simulink model "px4log"  (R2021a)
settings: Solver=FixedStepAuto  StartTime=0.0  StopTime=inf  RelTol=1e-3  EnableMultiTasking=on
model workspace (MAT data in the model file):
  Ts = 0.01
values from neighbouring files (symbols this model uses):
  den_lpf_d = den_lpf20    [Mainframe_init.m]    (also in load_autopilot.m)
  num_lpf_d = num_lpf20    [Mainframe_init.m]    (also in load_autopilot.m)
undefined symbols (not defined in the file or in its folder): Autopilot, AUX, dev, DiscIntNeverNeededParam, HIL_Data, pwm_output1, x, y, z
libraries: px4uORBlib x6, simulink_extras x4, px4Sensorslib x3, px4lib x2, simulink x1, sharedtransform x1
settings Model: SimulationMode=external  ExtModeTrigDuration=10  Creator=WrySi  LastModifiedBy=sasson
settings SolverCC: AlgebraicLoopSolver=TrustRegion  PositivePriorityOrder=on
settings DataIOCC: MaxDataPoints=2000
settings OptimizationCC: EnhancedBackFolding=on  PassReuseOutputArgsAs=Individual arguments  ZeroExternalMemoryAtStartup=off  ZeroInternalMemoryAtStartup=off  MaxStackSize=64  OptimizeBlockOrder=speed  DifferentSizesBufferReuse=on  OptimizationCustomize=off  EfficientTunableParamExpr=on
settings DebuggingCC: MultiTaskRateTransMsg=warning  ParameterOverflowMsg=none  ParameterTunabilityLossMsg=error  SymbolicDimsDataTypeCodeGenerationDiagnostic=none  SFMachineParentedDataDiag=warning
settings HardwareCC: ProdBitPerPointer=32  ProdBitPerSizeT=32  ProdBitPerPtrDiffT=32  ProdLargestAtomicInteger=Long  ProdLargestAtomicFloat=Double  ProdWordSize=32  ProdLongLongMode=on  ProdHWDeviceType=ARM Compatible->ARM Cortex
settings SFSimCC: MATLABDynamicMemAlloc=off  SimTargetLang=C++
settings RTWCC: SystemTargetFile=ert.tlc  HardwareBoard=PX4 Pixhawk 2.1 (Cube)  TLCOptions="-aInlineSetEventsForThisBaseRateFcn=TLC_FALSE -aSuppressMultiTaskScheduler=TLC_FALSE  -aRateBasedStepFcn=0"  TemplateMakefile=ert_default_tmf  GenerateReport=on  Toolchain=GNU Tools for PX4 Autopilots  IncludeHyperlinkInReport=on  LaunchReport=on  TargetLang=C++  GenerateTraceInfo=on  GenerateTraceReport=on  GenerateTraceReportSl=on  GenerateTraceReportSf=on  GenerateTraceReportEml=on
settings CodeAppCC: ForceParamTrailComments=on  IgnoreCustomStorageClasses=off  OperatorAnnotations=on  SimulinkDataObjDesc=on  SFDataObjDesc=on  InsertBlockDesc=on
settings ERTTargetCC: MatFileLogging=on  SupportContinuousTime=on  ExtMode=on  ExtModeMexArgs='127.0.0.1' 1 17725

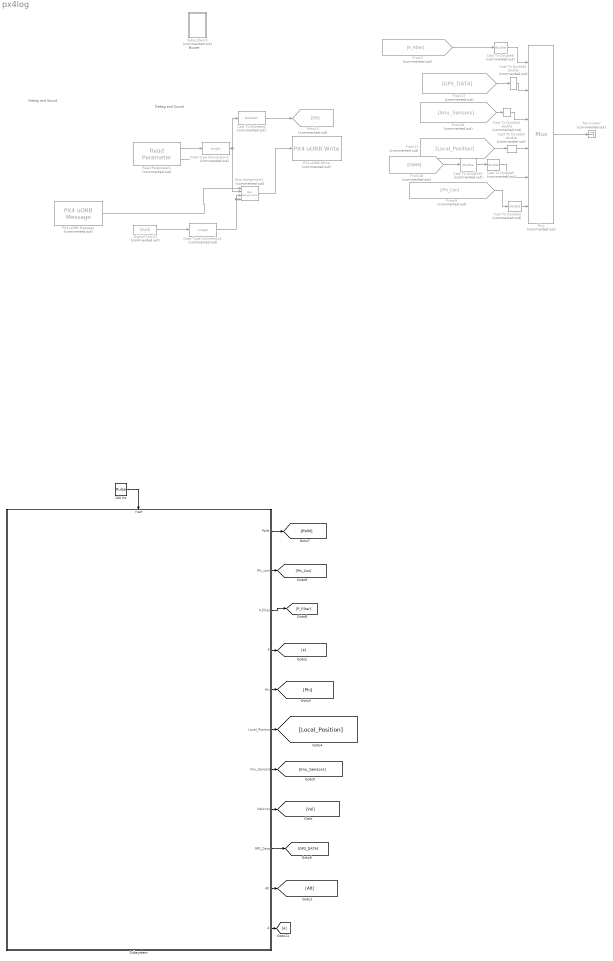
== system px4log ==
  note: Debag and Sound
  note: Debag and Sound
  note: Buzzer
  100 Hz : DiscretePulseGenerator  PulseType=Time based  Period=0.01  PulseWidth=50
  Bus Assignment1 : BusAssignment  Commented=on  AssignedSignals=x,z,y
  Cast To Boolean2 : DataTypeConversion  Commented=on  OutDataTypeStr=boolean
  Cast To Double{1..6,35} (7 alike) : DataTypeConversion  Commented=on  OutDataTypeStr=double
  Data Type Conversion1 : DataTypeConversion  Commented=on  OutDataTypeStr=single
  Data Type Conversion3 : DataTypeConversion  Commented=on  OutDataTypeStr=single
  Digital Clock2 : DigitalClock  Commented=on
  From11 : From  Commented=on  GotoTag=Local_Position
  From16 : From  Commented=on  GotoTag=Imu_Sensors
  From17 : From  Commented=on  GotoTag=GPS_DATA
  From18 : From  Commented=on  GotoTag=PWM
  From7 : From  Commented=on  GotoTag=P_Filter
  From9 : From  Commented=on  GotoTag=Phi_Con
  Goto10 : Goto  Commented=on  GotoTag=EN
  Mux : Mux  Commented=on  Inputs=6
  PX4 uORB Message : px4uORBlib/PX4 uORB Message  Commented=on  uORBTopic=debug_vect  SampleTime=1  selectInstance=debug_vect
      settings: SourceProductBaseCode=PX4AUTOPILOTS
  PX4 uORB Write : px4uORBlib/PX4 uORB Write  Commented=on  uORBTopic=debug_vect  selectInstance=debug_vect  MessageQueueLen=1
      settings: SourceProductBaseCode=PX4AUTOPILOTS
  Read Parameter1 : px4lib/Read Parameter  Commented=on  ParameterName=SD_save_flag  DataType=INT32  SampleTime=1
      settings: SourceProductBaseCode=PX4AUTOPILOTS
  Subsystem : Subsystem
  Subsystem3 : Subsystem  Commented=on
  Terminator : Terminator  Commented=on
  wires:
  Subsystem/7(Imu_Sensors) -> [Imu_Sensors]
  Subsystem/5(Phi) -> [Phi]
  Read Parameter1/1 -> Data Type Conversion3/1
  Bus Assignment1/1 -> PX4 uORB Write/1
  From9/1 -> Cast To Double4/1
  From17/1 -> Cast To Double1/1
  From16/1 -> Cast To Double2/1
  PX4 uORB Message/1 -> Bus Assignment1/1
  Data Type Conversion1/1 -> Bus Assignment1/3, Bus Assignment1/4
  From18/1 -> Cast To Double35/1
  Read Parameter1/2 -> ?
  Cast To Double35/1 -> Cast To Double5/1
  Subsystem/4(P) -> [P]
  100 Hz/1 -> Subsystem/Trigger
  Subsystem/9(GPS_Data) -> [GPS_DATA]
  Subsystem/2(Phi_com) -> [Phi_Con]
  Subsystem/3(P_filter) -> [P_Filter]
  Data Type Conversion3/1 -> Bus Assignment1/2, Cast To Boolean2/1
  Cast To Boolean2/1 -> Goto10/1
  Subsystem/10(Alt) -> [Alt]
  Subsystem/11(A) -> [A]
  Subsystem/6(Local_Position) -> [Local_Position]
  From11/1 -> Cast To Double3/1
  From7/1 -> Cast To Double6/1
  Subsystem/1(PWM) -> [PWM]
  Subsystem/8(Velocity) -> [Vel]
  Digital Clock2/1 -> Data Type Conversion1/1
  Mux/1 -> Terminator/1
  Cast To Double1/1 -> Mux/2
  Cast To Double2/1 -> Mux/3
  Cast To Double3/1 -> Mux/4
  Cast To Double4/1 -> Mux/6
  Cast To Double5/1 -> Mux/5
  Cast To Double6/1 -> Mux/1

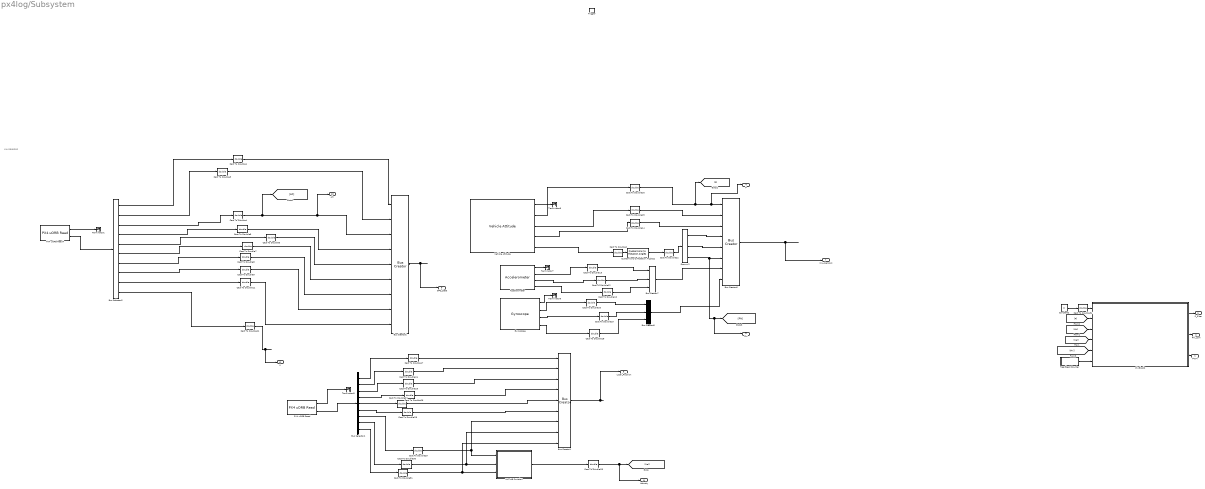
== system px4log/Subsystem ==
  note: IMU SENSORS
  Trigger : TriggerPort  VariantControl=Variant  PortDimensions=1
  Accelerometer : px4Sensorslib/Accelerometer  uorbTimeStamp=off  BlockingMode=off  BlockTimeout=1e-3  sampleTime=-1
      settings: SourceProductBaseCode=PX4AUTOPILOTS
  Bus Creator1 : BusCreator  Inputs=9
  Bus Creator2 : BusCreator  Inputs=9
  Bus Creator6 : BusCreator  Inputs=8
  Bus Creator7 : BusCreator  Inputs=3
  Bus Creator8 : BusCreator  Inputs=3
  Bus Selector1 : BusSelector  OutputSignals=ax,ay,az,z,x,y,vx,vy,vz
  Bus Selector2 : BusSelector  OutputSignals=lat,lon,alt,fix_type,satellites_used,vel_m_s,vel_n_m_s,vel_e_m_s,vel_d_m_s,timestamp
  Cast To Double{1..22,24..31,33..34} (32 alike) : DataTypeConversion  OutDataTypeStr=double
  Constant2 : Constant  Value=0  SampleTime=-1
  Demux2 : Demux  Outputs=3
  Gyroscope : px4Sensorslib/Gyroscope  uorbTimeStamp=off  BlockingMode=off  BlockTimeout=1e-3  sampleTime=-1
      settings: SourceProductBaseCode=PX4AUTOPILOTS
  Heartbeat Counter : Subsystem
  MATLAB Function : MATLAB Function  TreatAsAtomicUnit=on
  PX4 uORB Read : px4uORBlib/PX4 uORB Read  uORBTopic=vehicle_local_position  selectInstance=vehicle_local_position  SampleTime=-1  BlockingMode=off  BlockTimeout=1e-3
      settings: SourceProductBaseCode=PX4AUTOPILOTS
  PX4 uORB Read4 : px4uORBlib/PX4 uORB Read  uORBTopic=vehicle_gps_position  selectInstance=vehicle_gps_position  SampleTime=-1  BlockingMode=off  BlockTimeout=1e-3
      settings: SourceProductBaseCode=PX4AUTOPILOTS
  PixBlock2 : Subsystem
  Quaternions to Rotation Angles2 : sharedtransform/Quaternions to Rotation Angles  rotationOrder=ZYX  aMode=aMode
      settings: SourceProductBaseCode=AE,PW,DR,MT,UV,VE
  Terminator{1,3,7..9} (5 alike) : Terminator
  Vehicle Attitude : px4Sensorslib/Vehicle Attitude  rollRate=on  pitchRate=on  yawRate=on  quaternion=on  uorbTimeStamp=off  BlockingMode=off  BlockTimeout=0.001  sampleTime=-1
      settings: SourceProductBaseCode=PX4AUTOPILOTS
  PWM : Outport
  Phi_com : Outport  Port=2
  P_filter : Outport  Port=3
  P : Outport  Port=4
  Phi : Outport  Port=5
  Local_Position : Outport  Port=6
  Imu_Sensors : Outport  Port=7
  Velocity : Outport  Port=8
  GPS_Data : Outport  Port=9
  Alt : Outport  Port=10
  A : Outport  Port=11
  wires:
  Cast To Double27/1 -> Bus Creator1/5
  PX4 uORB Read/1 -> Terminator3/1
  Cast To Double22/1 -> Demux2/1
  Cast To Double31/1 -> Bus Creator1/9, MATLAB Function/3(vz)
  PX4 uORB Read/2 -> Bus Selector1/1
  Bus Selector2/7 -> Cast To Double8/1  "<vel_n_m_s>"
  PixBlock2/1(P_filter) -> P_filter/1
  Bus Creator8/1 -> Bus Creator6/8  "gyro"
  Bus Selector2/8 -> Cast To Double9/1  "<vel_e_m_s>"
  Cast To Double4/1 -> [Alt], Alt/1, Bus Creator2/3
  Bus Selector1/2 -> Cast To Double24/1  "<ay>"
  Cast To Double16/1 -> [P], P/1, Bus Creator6/1
  Gyroscope/4 -> Cast To Double18/1  "gyroZ"
  Bus Selector2/1 -> Cast To Double1/1  "<lat>"
  PX4 uORB Read4/1 -> Terminator1/1
  PixBlock2/3(PWM) -> PWM/1
  Cast To Double9/1 -> Bus Creator2/8
  Vehicle Attitude/2 -> Cast To Double16/1  "p"
  Cast To Double14/1 -> Bus Creator6/3
  [Alt] -> PixBlock2/3(Alt)
  Cast To Double24/1 -> Bus Creator1/2
  Vehicle Attitude/3 -> Cast To Double15/1  "q"
  Cast To Double33/1 -> [Vel], Velocity/1
  Demux2/3 -> [Phi], Phi/1, Bus Creator6/6  "phi"
  Cast To Double26/1 -> Bus Creator1/4
  Vehicle Attitude/4 -> Cast To Double14/1  "r"
  Bus Selector1/6 -> Cast To Double28/1  "<y>"
  Cast To Double17/1 -> Bus Creator1/1
  Cast To Double13/1 -> Bus Creator7/1
  Cast To Double20/1 -> Bus Creator8/1
  Cast To Double18/1 -> Bus Creator8/3
  Bus Selector2/3 -> Cast To Double4/1  "<alt>"
  Vehicle Attitude/5 -> Cast To Double2/1
  Bus Selector2/5 -> Cast To Double6/1  "<satellites_used>"
  Accelerometer/1 -> Terminator7/1
  Bus Selector1/5 -> Cast To Double27/1  "<x>"
  Cast To Double10/1 -> Bus Creator7/3
  Cast To Double1/1 -> Bus Creator2/1
  Cast To Double6/1 -> Bus Creator2/5
  Cast To Double25/1 -> Bus Creator1/3
  Cast To Double8/1 -> Bus Creator2/7
  Gyroscope/1 -> Terminator9/1
  Cast To Double28/1 -> Bus Creator1/6
  [Vel] -> PixBlock2/4(Velocity)
  Cast To Double5/1 -> Bus Creator2/4
  Bus Creator7/1 -> Bus Creator6/7  "accelerometer"
  Quaternions to Rotation Angles2/1 -> Cast To Double22/1  "euler from PX conj"
  Cast To Double29/1 -> Bus Creator1/7, MATLAB Function/1(vx)
  Bus Selector1/3 -> Cast To Double25/1  "<az>"
  Cast To Double15/1 -> Bus Creator6/2
  PixBlock2/2(Fin_cmd) -> Phi_com/1
  PX4 uORB Read4/2 -> Bus Selector2/1
  Cast To Double7/1 -> Bus Creator2/6
  Accelerometer/4 -> Cast To Double10/1  "accZ"
  Bus Selector2/4 -> Cast To Double5/1  "<fix_type>"
  Bus Selector2/9 -> Cast To Double11/1  "<vel_d_m_s>"
  Bus Selector1/7 -> Cast To Double29/1  "<vx>"
  Bus Selector1/1 -> Cast To Double17/1  "<ax>"
  Cast To Double2/1 -> Quaternions to Rotation Angles2/1
  Bus Selector1/9 -> Cast To Double31/1  "<vz>"
  Bus Creator2/1 -> GPS_Data/1
  Heartbeat Counter/1(Out1) -> PixBlock2/6(Heartbeat)  "send"
  Demux2/1 -> Bus Creator6/4  "psi"
  Bus Creator6/1 -> Imu_Sensors/1
  Cast To Double30/1 -> Bus Creator1/8, MATLAB Function/2(vy)
  Bus Selector1/8 -> Cast To Double30/1  "<vy>"
  Accelerometer/3 -> Cast To Double12/1  "accY"
  [P] -> PixBlock2/2(P_rms)
  [Phi] -> PixBlock2/5(Phi)
  Gyroscope/3 -> Cast To Double19/1  "gyroY"
  Gyroscope/2 -> Cast To Double20/1  "gyroX"
  Cast To Double3/1 -> Bus Creator2/2
  Cast To Double21/1 -> A/1
  Bus Selector2/2 -> Cast To Double3/1  "<lon>"
  Cast To Double34/1 -> PixBlock2/1(Phi_cmd)
  Accelerometer/2 -> Cast To Double13/1  "accX"
  Cast To Double11/1 -> Bus Creator2/9
  Constant2/1 -> Cast To Double34/1
  Cast To Double19/1 -> Bus Creator8/2
  Demux2/2 -> Bus Creator6/5  "theta"
  Bus Selector2/6 -> Cast To Double7/1  "<vel_m_s>"
  MATLAB Function/1(y) -> Cast To Double33/1
  Vehicle Attitude/1 -> Terminator8/1
  Cast To Double12/1 -> Bus Creator7/2
  Bus Selector1/4 -> Cast To Double26/1  "<z>"
  Bus Creator1/1 -> Local_Position/1
  Bus Selector2/10 -> Cast To Double21/1  "<timestamp>"

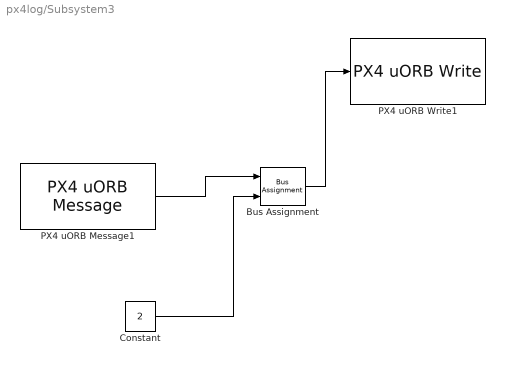
== system px4log/Subsystem3 ==
  Bus Assignment : BusAssignment  AssignedSignals=tune_id
  Constant : Constant  Value=2  OutDataTypeStr=uint8  SampleTime=60
  PX4 uORB Message1 : px4uORBlib/PX4 uORB Message  uORBTopic=tune_control  SampleTime=60  selectInstance=tune_control
      settings: SourceProductBaseCode=PX4AUTOPILOTS
  PX4 uORB Write1 : px4uORBlib/PX4 uORB Write  uORBTopic=tune_control  selectInstance=tune_control  MessageQueueLen=1
      settings: SourceProductBaseCode=PX4AUTOPILOTS
  wires:
  PX4 uORB Message1/1 -> Bus Assignment/1
  Bus Assignment/1 -> PX4 uORB Write1/1
  Constant/1 -> Bus Assignment/2

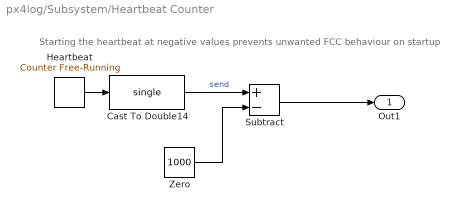
== system px4log/Subsystem/Heartbeat Counter ==
  note: Starting the heartbeat at negative values prevents unwanted FCC behaviour on startup
  Cast To Double14 : DataTypeConversion  OutDataTypeStr=single
  Heartbeat : simulink/Sources/Counter Free-Running  NumBits=16  tsamp=-1
  Subtract : Sum  Inputs=+-
  Zero : Constant  Value=1000  OutDataTypeStr=Inherit: Inherit via back propagation
  Out1 : Outport
  wires:
  Heartbeat/1 -> Cast To Double14/1
  Zero/1 -> Subtract/2
  Cast To Double14/1 -> Subtract/1  "send"
  Subtract/1 -> Out1/1

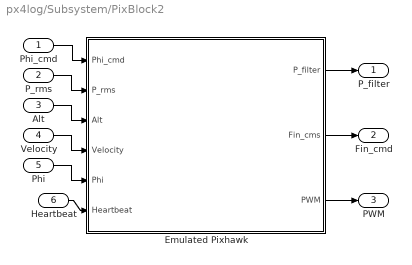
== system px4log/Subsystem/PixBlock2 ==
  Phi_cmd : Inport
  P_rms : Inport  Port=2
  Alt : Inport  Port=3
  Velocity : Inport  Port=4
  Phi : Inport  Port=5
  Heartbeat : Inport  Port=6
  Emulated Pixhawk : Subsystem
  P_filter : Outport
  Fin_cmd : Outport  Port=2
  PWM : Outport  Port=3
  wires:
  Emulated Pixhawk/1(P_filter) -> P_filter/1
  Phi_cmd/1 -> Emulated Pixhawk/1(Phi_cmd)
  P_rms/1 -> Emulated Pixhawk/2(P_rms)
  Phi/1 -> Emulated Pixhawk/5(Phi)
  Velocity/1 -> Emulated Pixhawk/4(Velocity)
  Alt/1 -> Emulated Pixhawk/3(Alt)
  Emulated Pixhawk/2(Fin_cms) -> Fin_cmd/1
  Heartbeat/1 -> Emulated Pixhawk/6(Heartbeat)
  Emulated Pixhawk/3(PWM) -> PWM/1

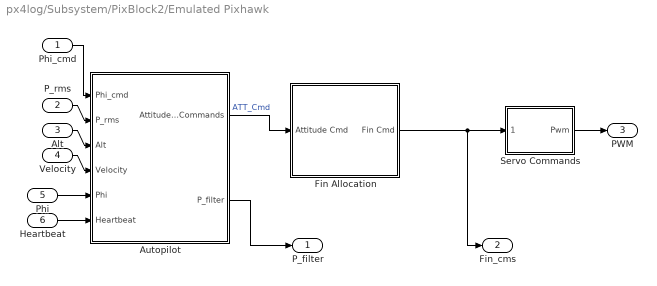
== system px4log/Subsystem/PixBlock2/Emulated Pixhawk ==
  Phi_cmd : Inport
  P_rms : Inport  Port=2
  Alt : Inport  Port=3
  Velocity : Inport  Port=4
  Phi : Inport  Port=5
  Heartbeat : Inport  Port=6
  Autopilot : Subsystem
  Fin Allocation : Subsystem
  Servo Commands : Subsystem
  P_filter : Outport  VectorParamsAs1DForOutWhenUnconnected=off
  Fin_cms : Outport  Port=2  VectorParamsAs1DForOutWhenUnconnected=off
  PWM : Outport  Port=3  VectorParamsAs1DForOutWhenUnconnected=off
  wires:
  Alt/1 -> Autopilot/3(Alt)
  Fin Allocation/1(Fin Cmd) -> Fin_cms/1, Servo Commands/1(Fin Cmd)
  Autopilot/1(Attitude_Commands) -> Fin Allocation/1(Attitude Cmd)  "ATT_Cmd"
  Phi_cmd/1 -> Autopilot/1(Phi_cmd)
  Velocity/1 -> Autopilot/4(Velocity)
  Phi/1 -> Autopilot/5(Phi)
  P_rms/1 -> Autopilot/2(P_rms)
  Autopilot/2(P_filter) -> P_filter/1
  Heartbeat/1 -> Autopilot/6(Heartbeat)
  Servo Commands/1(Pwm) -> PWM/1

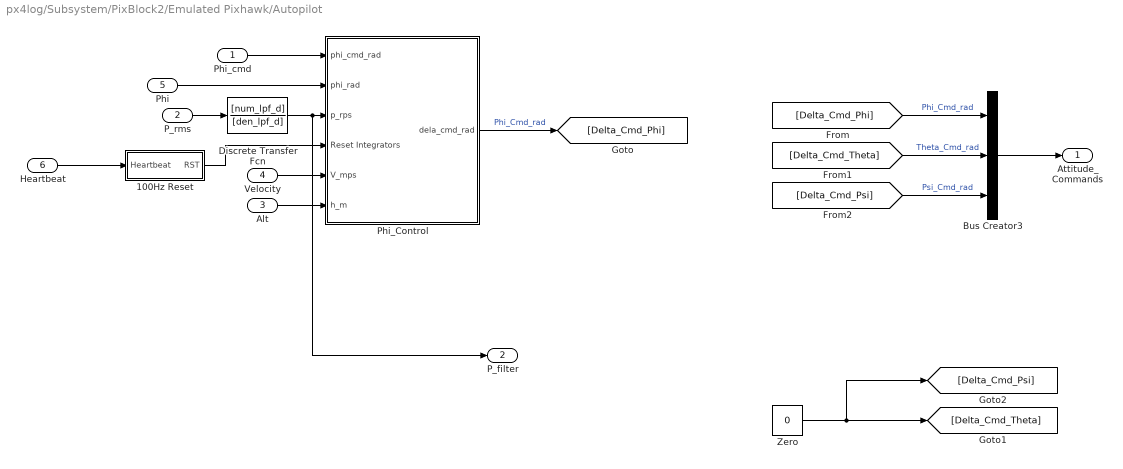
== system px4log/Subsystem/PixBlock2/Emulated Pixhawk/Autopilot ==
  Phi_cmd : Inport
  P_rms : Inport  Port=2
  Alt : Inport  Port=3
  Velocity : Inport  Port=4
  Phi : Inport  Port=5
  Heartbeat : Inport  Port=6
  100Hz Reset : Subsystem
  Bus Creator3 : BusCreator  Inputs=3
  Discrete Transfer Fcn : DiscreteTransferFcn  Numerator=[num_lpf_d]  Denominator=[den_lpf_d]
  Phi_Control : Subsystem
  Zero : Constant  Value=0  OutDataTypeStr=Inherit: Inherit via back propagation
  Attitude_Commands : Outport  VectorParamsAs1DForOutWhenUnconnected=off
  P_filter : Outport  Port=2  VectorParamsAs1DForOutWhenUnconnected=off
  wires:
  P_rms/1 -> Discrete Transfer Fcn/1
  Velocity/1 -> Phi_Control/5(V_mps)
  Zero/1 -> [Delta_Cmd_Psi], [Delta_Cmd_Theta]
  [Delta_Cmd_Phi] -> Bus Creator3/1  "Phi_Cmd_rad"
  [Delta_Cmd_Theta] -> Bus Creator3/2  "Theta_Cmd_rad"
  Bus Creator3/1 -> Attitude_Commands/1
  [Delta_Cmd_Psi] -> Bus Creator3/3  "Psi_Cmd_rad"
  100Hz Reset/1(RST) -> Phi_Control/4(Reset Integrators)
  Alt/1 -> Phi_Control/6(h_m)
  Phi_Control/1(dela_cmd_rad) -> [Delta_Cmd_Phi]  "Phi_Cmd_rad"
  Discrete Transfer Fcn/1 -> P_filter/1, Phi_Control/3(p_rps)
  Phi/1 -> Phi_Control/2(phi_rad)
  Heartbeat/1 -> 100Hz Reset/1(Heartbeat)
  Phi_cmd/1 -> Phi_Control/1(phi_cmd_rad)

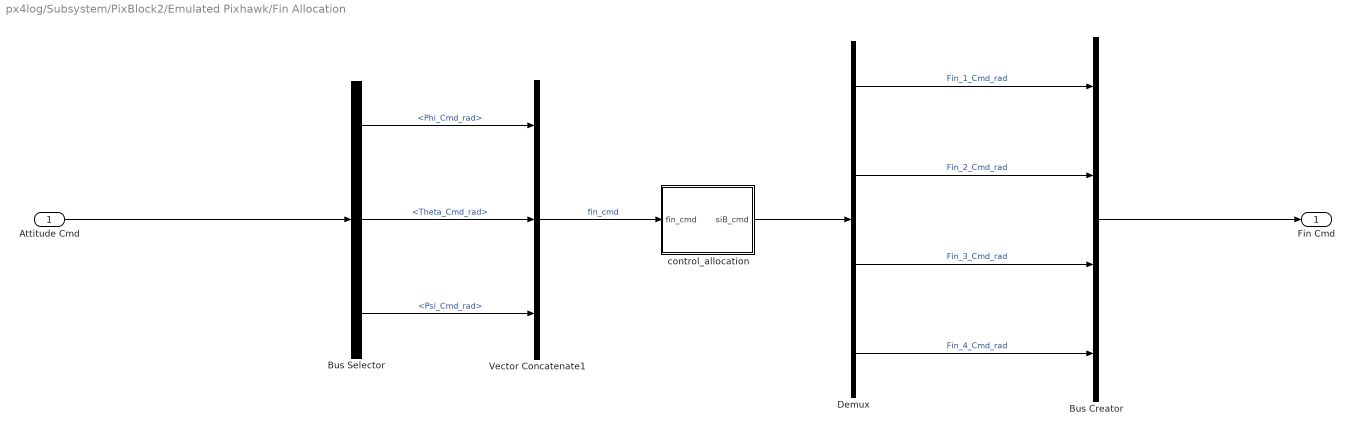
== system px4log/Subsystem/PixBlock2/Emulated Pixhawk/Fin Allocation ==
  Attitude Cmd : Inport
  Bus Creator : BusCreator  Inputs=4
  Bus Selector : BusSelector  OutputSignals=Phi_Cmd_rad,Theta_Cmd_rad,Psi_Cmd_rad
  Demux : Demux
  Vector Concatenate1 : Concatenate  NumInputs=3
  control_allocation : Subsystem
  Fin Cmd : Outport  VectorParamsAs1DForOutWhenUnconnected=off
  wires:
  Demux/4 -> Bus Creator/4  "Fin_4_Cmd_rad"
  control_allocation/1(siB_cmd) -> Demux/1
  Bus Selector/3 -> Vector Concatenate1/3  "<Psi_Cmd_rad>"
  Vector Concatenate1/1 -> control_allocation/1(fin_cmd)  "fin_cmd"
  Bus Selector/1 -> Vector Concatenate1/1  "<Phi_Cmd_rad>"
  Demux/3 -> Bus Creator/3  "Fin_3_Cmd_rad"
  Bus Selector/2 -> Vector Concatenate1/2  "<Theta_Cmd_rad>"
  Demux/1 -> Bus Creator/1  "Fin_1_Cmd_rad"
  Bus Creator/1 -> Fin Cmd/1
  Attitude Cmd/1 -> Bus Selector/1
  Demux/2 -> Bus Creator/2  "Fin_2_Cmd_rad"

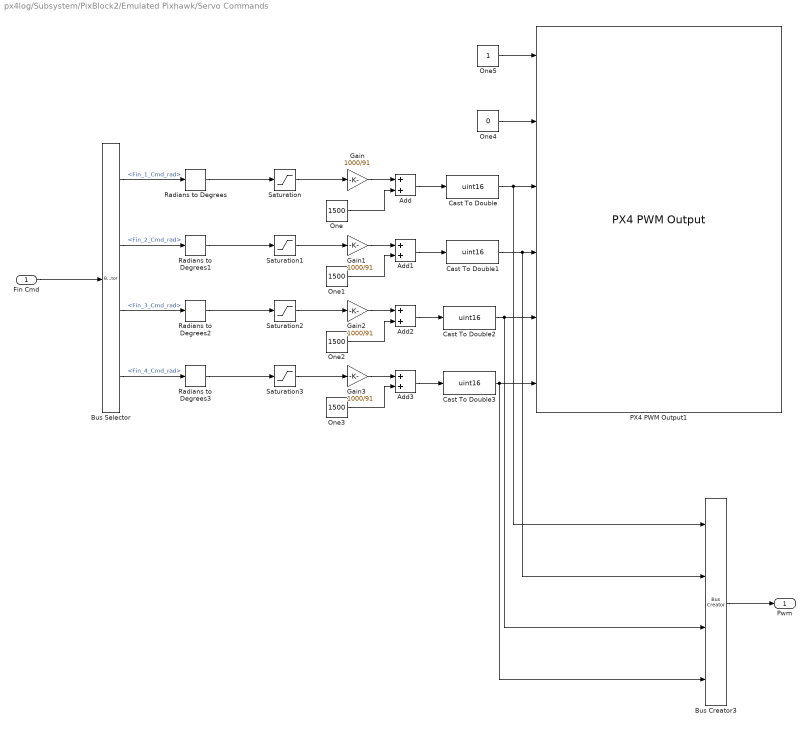
== system px4log/Subsystem/PixBlock2/Emulated Pixhawk/Servo Commands ==
  Fin Cmd : Inport
  Add{,1..3} (4 alike) : Sum
  Bus Creator3 : BusCreator  Inputs=4
  Bus Selector : BusSelector  OutputSignals=Fin_1_Cmd_rad,Fin_2_Cmd_rad,Fin_3_Cmd_rad,Fin_4_Cmd_rad
  Cast To Double{,1..3} (4 alike) : DataTypeConversion  OutDataTypeStr=uint16
  Gain{,1..3} (4 alike) : Gain  Gain=1000/91
  One{,1..3} (4 alike) : Constant  Value=1500  OutDataTypeStr=Inherit: Inherit via back propagation
  One4 : Constant  Value=0  OutDataTypeStr=boolean
  One5 : Constant  OutDataTypeStr=boolean
  PX4 PWM Output1 : px4lib/PX4 PWM Output  pwmDevice=AUX (/dev/pwm_output1)  pwmChannel1_=on  pwmChannel2_=on  pwmChannel3_=on  pwmChannel4_=on  pwmChannel5_=off  pwmChannel6_=off  pwmChannel7_=off  pwmChannel8_=off  forceTerminateFailsafe=off  outputErrorStatus=off
      settings: SourceProductBaseCode=PX4AUTOPILOTS
  Radians to Degrees{,1..3} (4 alike) : simulink_extras/Transformations/Radians to Degrees
  Saturation{,1..3} (4 alike) : Saturate  UpperLimit=20  LowerLimit=-20
  Pwm : Outport
  wires:
  Saturation2/1 -> Gain2/1
  One4/1 -> PX4 PWM Output1/2
  One/1 -> Add/2
  One2/1 -> Add2/2
  Add1/1 -> Cast To Double1/1
  Gain2/1 -> Add2/1
  Radians to Degrees1/1 -> Saturation1/1
  Add2/1 -> Cast To Double2/1
  Fin Cmd/1 -> Bus Selector/1
  Bus Selector/2 -> Radians to Degrees1/1  "<Fin_2_Cmd_rad>"
  Gain/1 -> Add/1
  Bus Selector/4 -> Radians to Degrees3/1  "<Fin_4_Cmd_rad>"
  One3/1 -> Add3/2
  Saturation/1 -> Gain/1
  Gain1/1 -> Add1/1
  Saturation3/1 -> Gain3/1
  Gain3/1 -> Add3/1
  Radians to Degrees3/1 -> Saturation3/1
  Bus Selector/1 -> Radians to Degrees/1  "<Fin_1_Cmd_rad>"
  Bus Selector/3 -> Radians to Degrees2/1  "<Fin_3_Cmd_rad>"
  Saturation1/1 -> Gain1/1
  Add3/1 -> Cast To Double3/1
  Radians to Degrees2/1 -> Saturation2/1
  Radians to Degrees/1 -> Saturation/1
  One1/1 -> Add1/2
  Add/1 -> Cast To Double/1
  Bus Creator3/1 -> Pwm/1
  Cast To Double/1 -> Bus Creator3/1, PX4 PWM Output1/3
  Cast To Double1/1 -> Bus Creator3/2, PX4 PWM Output1/4
  Cast To Double2/1 -> Bus Creator3/3, PX4 PWM Output1/5
  Cast To Double3/1 -> Bus Creator3/4, PX4 PWM Output1/6
  One5/1 -> PX4 PWM Output1/1

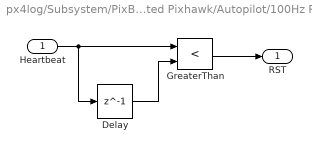
== system px4log/Subsystem/PixBlock2/Emulated Pixhawk/Autopilot/100Hz Reset ==
  Heartbeat : Inport
  Delay : Delay  DelayLength=1
  GreaterThan : RelationalOperator  Operator=<  OutDataTypeStr=boolean  RndMeth=Simplest
  RST : Outport
  wires:
  GreaterThan/1 -> RST/1
  Delay/1 -> GreaterThan/2
  Heartbeat/1 -> Delay/1, GreaterThan/1

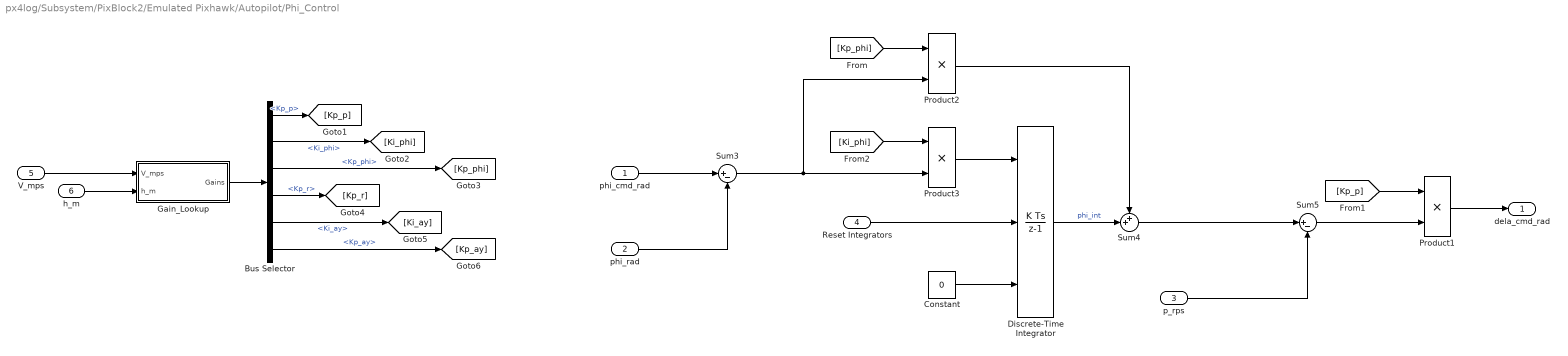
== system px4log/Subsystem/PixBlock2/Emulated Pixhawk/Autopilot/Phi_Control ==
  phi_cmd_rad : Inport
  phi_rad : Inport  Port=2
  p_rps : Inport  Port=3
  Reset Integrators : Inport  Port=4
  V_mps : Inport  Port=5
  h_m : Inport  Port=6
  Bus Selector : BusSelector  OutputSignals=Kp_p,Ki_phi,Kp_phi,Kp_r,Ki_ay,Kp_ay
  Constant : Constant  Value=0  OutDataTypeStr=single
  Discrete-Time Integrator : DiscreteIntegrator  ExternalReset=level  InitialConditionSource=external  SampleTime=-1  OutDataTypeStr=single  ICPrevOutput=DiscIntNeverNeededParam  ICPrevScaledInput=DiscIntNeverNeededParam
  Gain_Lookup : Subsystem
  Product1 : Product
  Product2 : Product
  Product3 : Product
  Sum3 : Sum  Inputs=|+-
  Sum4 : Sum  Inputs=++|
  Sum5 : Sum  Inputs=|+-
  dela_cmd_rad : Outport
  wires:
  phi_cmd_rad/1 -> Sum3/1
  Reset Integrators/1 -> Discrete-Time Integrator/2
  p_rps/1 -> Sum5/2
  phi_rad/1 -> Sum3/2
  Product2/1 -> Sum4/1
  Sum3/1 -> Product3/2, Product2/2
  Constant/1 -> Discrete-Time Integrator/3
  Sum5/1 -> Product1/2
  [Ki_phi] -> Product3/1
  Product1/1 -> dela_cmd_rad/1
  [Kp_p] -> Product1/1
  [Kp_phi] -> Product2/1
  Discrete-Time Integrator/1 -> Sum4/2  "phi_int"
  Sum4/1 -> Sum5/1
  Product3/1 -> Discrete-Time Integrator/1
  h_m/1 -> Gain_Lookup/2(h_m)
  Bus Selector/6 -> [Kp_ay]  "<Kp_ay>"
  Bus Selector/5 -> [Ki_ay]  "<Ki_ay>"
  Bus Selector/2 -> [Ki_phi]  "<Ki_phi>"
  Bus Selector/1 -> [Kp_p]  "<Kp_p>"
  V_mps/1 -> Gain_Lookup/1(V_mps)
  Bus Selector/4 -> [Kp_r]  "<Kp_r>"
  Gain_Lookup/1(Gains) -> Bus Selector/1
  Bus Selector/3 -> [Kp_phi]  "<Kp_phi>"

== system px4log/Subsystem/PixBlock2/Emulated Pixhawk/Fin Allocation/control_allocation ==
  fin_cmd : Inport
  Constant7 : Constant  Value=HIL_Data.FDM.Tr4r3  OutDataTypeStr=single
  Product : Product  Multiplication=Matrix(*)
  siB_cmd : Outport  VectorParamsAs1DForOutWhenUnconnected=off
  wires:
  Constant7/1 -> Product/1
  fin_cmd/1 -> Product/2
  Product/1 -> siB_cmd/1  "siB_cmd"

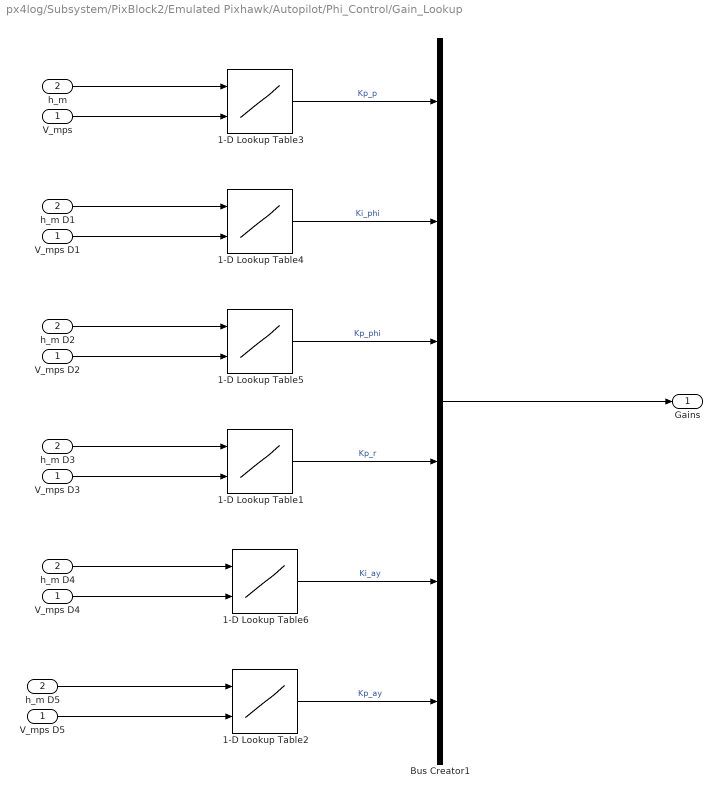
== system px4log/Subsystem/PixBlock2/Emulated Pixhawk/Autopilot/Phi_Control/Gain_Lookup ==
  V_mps : Inport
  h_m : Inport  Port=2
  1-D Lookup Table1 : Lookup_n-D  BreakpointsForDimension1=Autopilot.Ay.h_bkpts_m  BreakpointsForDimension2=Autopilot.Ay.V_bkpts_mps  Table=Autopilot.Ay.Kp_r_vec  ExtrapMethod=Clip  UseLastTableValue=on  InternalRulePriority=Speed  RndMeth=Simplest  InputSameDT=on
      settings: InputPortMap=u0,u1
      settings: AttributesFormatString=|
      | %<Table>
      | %<BreakpointsForDimension1>
      | %<BreakpointsForDimension2>
  1-D Lookup Table2 : Lookup_n-D  BreakpointsForDimension1=Autopilot.Ay.h_bkpts_m  BreakpointsForDimension2=Autopilot.Ay.V_bkpts_mps  Table=Autopilot.Ay.Kp_ay_vec  ExtrapMethod=Clip  UseLastTableValue=on  InternalRulePriority=Speed  RndMeth=Simplest  InputSameDT=on
      settings: InputPortMap=u0,u1
      settings: AttributesFormatString=|
      | %<Table>
      | %<BreakpointsForDimension1>
      | %<BreakpointsForDimension2>
  1-D Lookup Table3 : Lookup_n-D  BreakpointsForDimension1=Autopilot.Phi.h_bkpts_m  BreakpointsForDimension2=Autopilot.Phi.V_bkpts_mps  Table=Autopilot.Phi.Kp_p_vec  ExtrapMethod=Clip  UseLastTableValue=on  InternalRulePriority=Speed  RndMeth=Simplest  InputSameDT=on
      settings: InputPortMap=u0,u1
      settings: AttributesFormatString=|
      | %<Table>
      | %<BreakpointsForDimension1>
      | %<BreakpointsForDimension2>
  1-D Lookup Table4 : Lookup_n-D  BreakpointsForDimension1=Autopilot.Phi.h_bkpts_m  BreakpointsForDimension2=Autopilot.Phi.V_bkpts_mps  Table=Autopilot.Phi.Ki_phi_vec  ExtrapMethod=Clip  UseLastTableValue=on  InternalRulePriority=Speed  RndMeth=Simplest  InputSameDT=on
      settings: InputPortMap=u0,u1
      settings: AttributesFormatString=|
      | %<Table>
      | %<BreakpointsForDimension1>
      | %<BreakpointsForDimension2>
  1-D Lookup Table5 : Lookup_n-D  BreakpointsForDimension1=Autopilot.Phi.h_bkpts_m  BreakpointsForDimension2=Autopilot.Phi.V_bkpts_mps  Table=Autopilot.Phi.Kp_phi_vec  ExtrapMethod=Clip  UseLastTableValue=on  InternalRulePriority=Speed  RndMeth=Simplest  InputSameDT=on
      settings: InputPortMap=u0,u1
      settings: AttributesFormatString=|
      | %<Table>
      | %<BreakpointsForDimension1>
      | %<BreakpointsForDimension2>
  1-D Lookup Table6 : Lookup_n-D  BreakpointsForDimension1=Autopilot.Ay.h_bkpts_m  BreakpointsForDimension2=Autopilot.Ay.V_bkpts_mps  Table=Autopilot.Ay.Ki_ay_vec  ExtrapMethod=Clip  UseLastTableValue=on  InternalRulePriority=Speed  RndMeth=Simplest  InputSameDT=on
      settings: InputPortMap=u0,u1
      settings: AttributesFormatString=|
      | %<Table>
      | %<BreakpointsForDimension1>
      | %<BreakpointsForDimension2>
  Bus Creator1 : BusCreator  Inputs=6
  V_mps D{1..5} (5 alike) : InportShadow
  h_m D{1..5} (5 alike) : InportShadow  Port=2
  Gains : Outport
  wires:
  h_m/1 -> 1-D Lookup Table3/1
  Bus Creator1/1 -> Gains/1
  1-D Lookup Table5/1 -> Bus Creator1/3  "Kp_phi"
  1-D Lookup Table4/1 -> Bus Creator1/2  "Ki_phi"
  1-D Lookup Table3/1 -> Bus Creator1/1  "Kp_p"
  V_mps/1 -> 1-D Lookup Table3/2
  h_m D1/1 -> 1-D Lookup Table4/1
  V_mps D1/1 -> 1-D Lookup Table4/2
  h_m D2/1 -> 1-D Lookup Table5/1
  V_mps D2/1 -> 1-D Lookup Table5/2
  1-D Lookup Table2/1 -> Bus Creator1/6  "Kp_ay"
  1-D Lookup Table6/1 -> Bus Creator1/5  "Ki_ay"
  1-D Lookup Table1/1 -> Bus Creator1/4  "Kp_r"
  h_m D3/1 -> 1-D Lookup Table1/1
  V_mps D3/1 -> 1-D Lookup Table1/2
  h_m D4/1 -> 1-D Lookup Table6/1
  V_mps D4/1 -> 1-D Lookup Table6/2
  h_m D5/1 -> 1-D Lookup Table2/1
  V_mps D5/1 -> 1-D Lookup Table2/2

== matlab function px4log/Subsystem/MATLAB Function ==
  data: vx input; y output; vy input; vz input
function y = fcn(vx,vy,vz)

y = double(norm([vx vy vz]));
end
